simulink model "Citation"  (Simulink 10.1)
settings: Solver=ode5  StartTime=0.0  StopTime=inf  FixedStep=0.01  RelTol=1e-3  EnableMultiTasking=on
values from neighbouring files (symbols this model uses):
  S = 12.9900    (= 12.99)    [FTFC.m]
  Vw915 = 0    [initcit.m]
  winddir = 45*(pi/180)    (= 0.785398163397)    [initcit.m]
  x0 = []    [cessnac550_3d_sfnc.m]    (also in sfunxyz.m)
undefined symbols (not defined in the file or in its folder): chord, cv1, cv2, cv3, cv4, deltagmax1, deltagmax2, deltagmax3, deltagmax4, Deng, ealphag, ealphas, g0, hDME, hGS, kt1, kt2, kt3, lh, massinit, matbuaf, matdaf, matdam, matdbbf, matdeaf, matdgaf, matdqaf, matduaf, matdwaw, matedhr, mateif, matelhr, matemhr, matemv1, matemv2, matemve, matetam, mateuaf, matfaaf, matfaxl, matff, matibaf, matibmh, matipaf, matipmh, matiraf, matiuaf, matiwaf, matlaf, matlam, matleaf, matleam, matlgaf, matlqaf, matluaf, matmaaf, matmaam, matmaf, matmam, matmbbf ... (+74)
undefined symbols (not defined in the file): matibb
libraries: simulink x12, vrlib x1
(part 3 of 5)

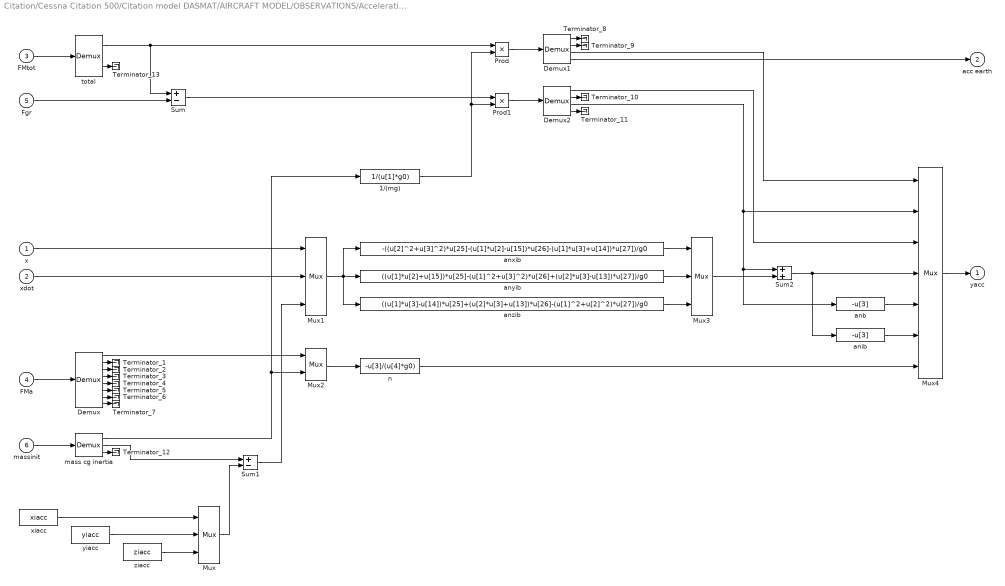
== system Citation/Cessna Citation 500/Citation model DASMAT/AIRCRAFT MODEL/OBSERVATIONS/Acceleration ==
  x : Inport
  xdot : Inport  Port=2
  FMtot : Inport  Port=3
  FMa : Inport  Port=4
  Fgr : Inport  Port=5
  massinit : Inport  Port=6
  1/(mg) : Fcn  Expr=1/(u[1]*g0)
  Demux : Demux  Outputs=[3 3 3 3 3 3 3 3]
      settings: DisplayOption=none
  Demux1 : Demux  Outputs=[3 3 3 3]
      settings: DisplayOption=none
  Demux2 : Demux  Outputs=[3 3 3 3]
      settings: DisplayOption=none
  Mux : Mux  Inputs=3
  Mux1 : Mux  Inputs=[12 12 3]
  Mux2 : Mux  Inputs=[3 1]
  Mux3 : Mux  Inputs=3
  Mux4 : Mux  Inputs=[3 3 3 3 1 1 1]
  Prod : Product  InputSameDT=on  SaturateOnIntegerOverflow=on  OutDataTypeStr=Inherit: Same as first input
  Prod1 : Product  InputSameDT=on  SaturateOnIntegerOverflow=on  OutDataTypeStr=Inherit: Same as first input
  Sum : Sum  Inputs=+-  InputSameDT=on  SaturateOnIntegerOverflow=on  OutDataTypeStr=Inherit: Same as first input
  Sum1 : Sum  Inputs=+-  InputSameDT=on  SaturateOnIntegerOverflow=on  OutDataTypeStr=Inherit: Same as first input
  Sum2 : Sum  InputSameDT=on  SaturateOnIntegerOverflow=on  OutDataTypeStr=Inherit: Same as first input
  Terminator_{1..13} (13 alike) : Terminator
  anb : Fcn  Expr=-u[3]
  anib : Fcn  Expr=-u[3]
  anxib : Fcn  Expr=-((u[2]^2+u[3]^2)*u[25]-(u[1]*u[2]-u[15])*u[26]-(u[1]*u[3]+u[14])*u[27])/g0
  anyib : Fcn  Expr=((u[1]*u[2]+u[15])*u[25]-(u[1]^2+u[3]^2)*u[26]+(u[2]*u[3]-u[13])*u[27])/g0
  anzib : Fcn  Expr=((u[1]*u[3]-u[14])*u[25]+(u[2]*u[3]+u[13])*u[26]-(u[1]^2+u[2]^2)*u[27])/g0
  mass cg inertia : Demux  Outputs=[1 3 4]
      settings: DisplayOption=none
  n : Fcn  Expr=-u[3]/(u[4]*g0)
  total : Demux  Outputs=[12 12]
      settings: DisplayOption=none
  xiacc : Constant  Value=xiacc
  yiacc : Constant  Value=yiacc
  ziacc : Constant  Value=ziacc
  yacc : Outport
  acc earth : Outport  Port=2
  wires:
  total/2 -> Terminator_13/1
  mass cg inertia/3 -> Terminator_12/1
  Demux2/4 -> Terminator_11/1
  Demux2/2 -> Terminator_10/1
  Demux1/2 -> Terminator_9/1
  Demux1/1 -> Terminator_8/1
  Demux/8 -> Terminator_7/1
  Demux/7 -> Terminator_6/1
  Demux/6 -> Terminator_5/1
  Demux/5 -> Terminator_4/1
  Demux/4 -> Terminator_3/1
  Demux/3 -> Terminator_2/1
  Demux/2 -> Terminator_1/1
  Mux4/1 -> yacc/1
  anb/1 -> Mux4/5
  Sum1/1 -> Mux1/3
  x/1 -> Mux1/1
  xdot/1 -> Mux1/2
  mass cg inertia/2 -> Sum1/1
  anzib/1 -> Mux3/3
  anxib/1 -> Mux3/1
  anyib/1 -> Mux3/2
  Mux2/1 -> n/1
  massinit/1 -> mass cg inertia/1
  xiacc/1 -> Mux/1
  yiacc/1 -> Mux/2
  ziacc/1 -> Mux/3
  1/(mg)/1 -> Prod1/2, Prod/2
  Sum/1 -> Prod1/1
  Mux1/1 -> anxib/1, anzib/1, anyib/1
  mass cg inertia/1 -> Mux2/2, 1/(mg)/1
  Mux/1 -> Sum1/2
  Mux3/1 -> Sum2/2
  Sum2/1 -> anib/1, Mux4/4
  FMa/1 -> Demux/1
  Fgr/1 -> Sum/2
  anib/1 -> Mux4/6
  n/1 -> Mux4/7
  total/1 -> Sum/1, Prod/1
  FMtot/1 -> total/1
  Demux/1 -> Mux2/1
  Demux2/3 -> Mux4/2, Sum2/1, anb/1
  Demux1/3 -> Mux4/1
  Prod/1 -> Demux1/1
  Demux2/1 -> Mux4/3
  Prod1/1 -> Demux2/1
  Demux1/4 -> acc earth/1

== system Citation/Cessna Citation 500/Citation model DASMAT/AIRCRAFT MODEL/OBSERVATIONS/Energy ==
  x : Inport
  xdot : Inport  Port=2
  yatm : Inport  Port=3
  Mux : Mux  Inputs=[12 12 8]
  Mux1 : Mux  Inputs=2
  spec energy : Fcn  Expr=u[10]+(u[4]*u[4])/(2*u[28])
  spec power : Fcn  Expr=u[22]+(u[4]*u[16])/u[28]
  ys : Outport
  wires:
  spec power/1 -> Mux1/2
  spec energy/1 -> Mux1/1
  x/1 -> Mux/1
  xdot/1 -> Mux/2
  Mux1/1 -> ys/1
  yatm/1 -> Mux/3
  Mux/1 -> spec power/1, spec energy/1

== system Citation/Cessna Citation 500/Citation model DASMAT/AIRCRAFT MODEL/OBSERVATIONS/Flight-Path ==
  x : Inport
  xdot : Inport  Port=2
  yuvw : Inport  Port=3
  acc earth : Inport  Port=4
  Demux : Demux  Outputs=[3 3 3 3]
      settings: DisplayOption=none
  Mux : Mux  Inputs=[12 12 3 3]
  Mux1 : Mux  Inputs=[30 1 1]
  Mux2 : Mux  Inputs=17
  Terminator11 : Terminator
  Terminator12 : Terminator
  Terminator13 : Terminator
  Vground : Fcn  Expr=sqrt(u[23]*u[23]+u[24]*u[24]+u[22]*u[22])
  bank angle : Fcn  Expr=asin(sin(u[7])*cos(u[8]))
  chi : Fcn  Expr=atan2(u[26],u[25])
  chidot : Fcn  Expr=(u[25]*u[29]*g0-u[28]*g0*u[26])/(u[4]*u[4]-u[27]*u[27])
  chimagn : Fcn  Expr=0
  chitrue : Fcn  Expr=atan2(u[24],u[23])
  chitruedot : Fcn  Expr=(u[23]*u[29]*g0-u[28]*g0*u[24])/(u[31]*u[31]-u[22]*u[22])
  flightpath acc : Fcn  Expr=u[16]/g0
  gamma : Fcn  Expr=asin(-u[27]/u[4])
  gammadot : Fcn  Expr=(-u[4]*u[30]*g0+u[16]*u[27])/(u[4]*sqrt(u[4]*u[4]-u[27]*u[27]))
  gammatrue : Fcn  Expr=asin(u[22]/u[31])
  gammatruedot : Fcn  Expr=(u[31]*u[32]*g0-u[16]*u[22])/(u[31]*sqrt(u[31]*u[31]-u[22]*u[22]))
  gsdev : Fcn  Expr=atan2(u[10]-hGS,sqrt((xGS-u[11])*(xGS-u[11])+(yGS-u[12])*(yGS-u[12]))) - 3*pi/180
  locdev : Fcn  Expr=psiLOC - atan2(yLOC-u[12],xLOC-u[11])
  psimagn : Fcn  Expr=0
  range : Fcn  Expr=sqrt((u[11]-xDME)*(u[11]-xDME)+(u[12]-yDME)*(u[12]-yDME)+(u[10]-hDME)*(u[10]-hDME))
  vertical acc : Fcn  Expr=-u[30]
  yfp : Outport
  wires:
  Demux/3 -> Terminator13/1
  Demux/2 -> Terminator12/1
  Demux/1 -> Terminator11/1
  vertical acc/1 -> Mux1/3, Mux2/16
  Mux1/1 -> gammatruedot/1, chitruedot/1, gammatrue/1, chitrue/1
  Vground/1 -> Mux1/2, Mux2/15
  xdot/1 -> Mux/2
  Demux/4 -> Mux/3
  acc earth/1 -> Mux/4
  yuvw/1 -> Demux/1
  chi/1 -> Mux2/2
  Mux2/1 -> yfp/1
  gamma/1 -> Mux2/1
  gammadot/1 -> Mux2/3
  chidot/1 -> Mux2/4
  gammatrue/1 -> Mux2/5
  chitrue/1 -> Mux2/6
  gammatruedot/1 -> Mux2/7
  flightpath acc/1 -> Mux2/17
  range/1 -> Mux2/14
  locdev/1 -> Mux2/13
  gsdev/1 -> Mux2/12
  bank angle/1 -> Mux2/11
  psimagn/1 -> Mux2/10
  chimagn/1 -> Mux2/9
  chitruedot/1 -> Mux2/8
  x/1 -> Mux/1
  Mux/1 -> Mux1/1, gammadot/1, chi/1, gamma/1, chidot/1, gsdev/1, locdev/1, range/1, Vground/1, vertical acc/1, flightpath acc/1, bank angle/1, psimagn/1, chimagn/1

== system Citation/Cessna Citation 500/Citation model DASMAT/AIRCRAFT MODEL/WIND/TURBULENCE/Logarithmic Wind model ==
  In1 : Inport
  He Selector : Selector  InputPortWidth=12  IndexOptions=Index vector (dialog)  Indices=[10]  OutputSizes=1
  Logarithmic Wind model : Subsystem
  Mux : Mux  Inputs=3
  Out1 : Outport
  wires:
  In1/1 -> He Selector/1
  Mux/1 -> Out1/1
  Logarithmic Wind model/1(uwind) -> Mux/1  "uwind"
  Logarithmic Wind model/2(vwind) -> Mux/2  "vwind"
  Logarithmic Wind model/3(wwind) -> Mux/3  "wwind"
  He Selector/1 -> Logarithmic Wind model/1(he)

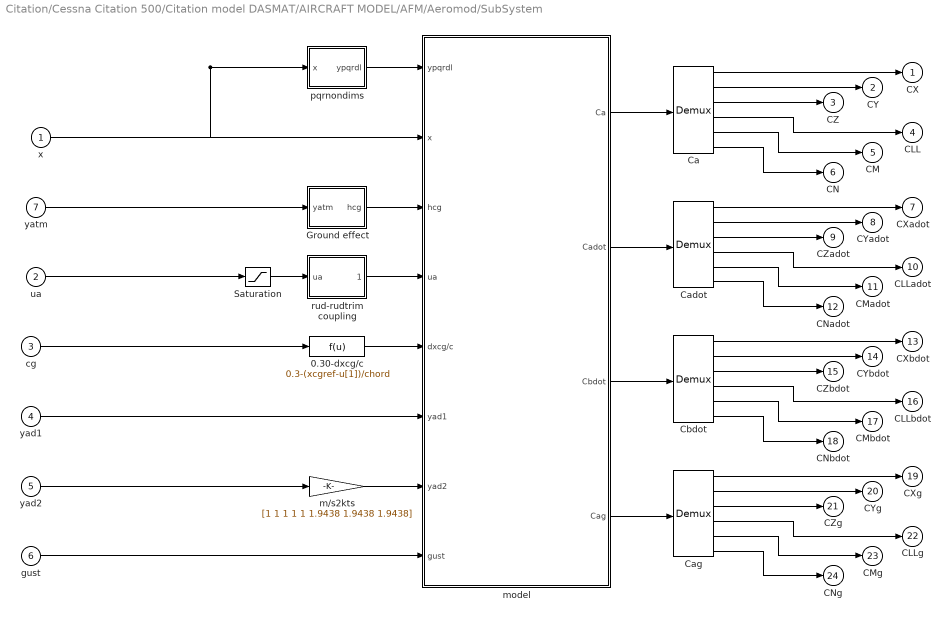
== system Citation/Cessna Citation 500/Citation model DASMAT/AIRCRAFT MODEL/AFM/Aeromod/SubSystem ==
  x : Inport
  ua : Inport  Port=2
  cg : Inport  Port=3
  yad1 : Inport  Port=4
  yad2 : Inport  Port=5
  gust : Inport  Port=6
  yatm : Inport  Port=7
  0.30-dxcg/c : Fcn  Expr=0.3-(xcgref-u[1])/chord
  Ca : Demux  Outputs=6
      settings: DisplayOption=none
  Cadot : Demux  Outputs=6
      settings: DisplayOption=none
  Cag : Demux  Outputs=6
      settings: DisplayOption=none
  Cbdot : Demux  Outputs=6
      settings: DisplayOption=none
  Ground effect : Subsystem
  Saturation : Saturate  UpperLimit="[ 15  37  22  15  20  10 40 180/pi]*pi/180"  LowerLimit="[-20 -37 -22 -15 -20 -10 0  0]*pi/180"
  m/s2kts : Gain  Gain=[1 1 1 1 1 1.9438 1.9438 1.9438]  SaturateOnIntegerOverflow=on  OutDataTypeStr=Inherit: Same as input  ParamDataTypeStr=Inherit: Same as input
  model : Subsystem
  pqrnondims : Subsystem
  rud-rudtrim coupling : Subsystem
  CX : Outport
  CY : Outport  Port=2
  CZ : Outport  Port=3
  CLL : Outport  Port=4
  CM : Outport  Port=5
  CN : Outport  Port=6
  CXadot : Outport  Port=7
  CYadot : Outport  Port=8
  CZadot : Outport  Port=9
  CLLadot : Outport  Port=10
  CMadot : Outport  Port=11
  CNadot : Outport  Port=12
  CXbdot : Outport  Port=13
  CYbdot : Outport  Port=14
  CZbdot : Outport  Port=15
  CLLbdot : Outport  Port=16
  CMbdot : Outport  Port=17
  CNbdot : Outport  Port=18
  CXg : Outport  Port=19
  CYg : Outport  Port=20
  CZg : Outport  Port=21
  CLLg : Outport  Port=22
  CMg : Outport  Port=23
  CNg : Outport  Port=24
  wires:
  yad2/1 -> m/s2kts/1
  m/s2kts/1 -> model/7(yad2)
  Saturation/1 -> rud-rudtrim coupling/1(ua)
  model/4(Cag) -> Cag/1
  model/3(Cbdot) -> Cbdot/1
  Cbdot/2 -> CYbdot/1
  Cbdot/1 -> CXbdot/1
  Cbdot/3 -> CZbdot/1
  Cbdot/4 -> CLLbdot/1
  Cbdot/5 -> CMbdot/1
  Cbdot/6 -> CNbdot/1
  Cag/6 -> CNg/1
  Cag/5 -> CMg/1
  Cag/4 -> CLLg/1
  Cag/3 -> CZg/1
  Cag/1 -> CXg/1
  Cag/2 -> CYg/1
  model/2(Cadot) -> Cadot/1
  Cadot/2 -> CYadot/1
  Cadot/1 -> CXadot/1
  Cadot/3 -> CZadot/1
  Cadot/4 -> CLLadot/1
  Cadot/5 -> CMadot/1
  Cadot/6 -> CNadot/1
  Ca/6 -> CN/1
  Ca/5 -> CM/1
  Ca/4 -> CLL/1
  Ca/3 -> CZ/1
  Ca/1 -> CX/1
  Ca/2 -> CY/1
  model/1(Ca) -> Ca/1
  yad1/1 -> model/6(yad1)
  gust/1 -> model/8(gust)
  cg/1 -> 0.30-dxcg/c/1
  ua/1 -> Saturation/1
  x/1 -> pqrnondims/1(x), model/2(x)
  0.30-dxcg/c/1 -> model/5(dxcg/c)
  Ground effect/1(hcg) -> model/3(hcg)
  rud-rudtrim coupling/1(ua coupled) -> model/4(ua)
  pqrnondims/1(ypqrdl) -> model/1(ypqrdl)
  yatm/1 -> Ground effect/1(yatm)

== system Citation/Cessna Citation 500/Citation model DASMAT/AIRCRAFT MODEL/AFM/FMaerodims/dims ==
  note: X,Y,Z
  FM/length : Inport
  Demux : Demux  Outputs=[12 3 3 3 3]
      settings: DisplayOption=none
  LL,M,N air : Gain  Gain=[span chord span]  SaturateOnIntegerOverflow=on  OutDataTypeStr=Inherit: Same as input  ParamDataTypeStr=Inherit: Same as input
  LL,M,N body : Gain  Gain=[span chord span]  SaturateOnIntegerOverflow=on  OutDataTypeStr=Inherit: Same as input  ParamDataTypeStr=Inherit: Same as input
  LL,M,N earth : Gain  Gain=[span chord span]  SaturateOnIntegerOverflow=on  OutDataTypeStr=Inherit: Same as input  ParamDataTypeStr=Inherit: Same as input
  LL,M,N stab : Gain  Gain=[span chord span]  SaturateOnIntegerOverflow=on  OutDataTypeStr=Inherit: Same as input  ParamDataTypeStr=Inherit: Same as input
  Mux : Mux  Inputs=[12 3 3 3 3]
  FM : Outport
  wires:
  LL,M,N earth/1 -> Mux/5
  Demux/5 -> LL,M,N earth/1
  LL,M,N body/1 -> Mux/4
  LL,M,N stab/1 -> Mux/3
  LL,M,N air/1 -> Mux/2
  Demux/1 -> Mux/1
  Demux/2 -> LL,M,N air/1
  Demux/3 -> LL,M,N stab/1
  Demux/4 -> LL,M,N body/1
  Mux/1 -> FM/1
  FM/length/1 -> Demux/1

== system Citation/Cessna Citation 500/Citation model DASMAT/AIRCRAFT MODEL/AFM/FMaerodims/dims1 ==
  note: X,Y,Z
  F FM/length : Inport
  Demux : Demux  Outputs=[12 3 3 3 3]
      settings: DisplayOption=none
  LL,M,N air : Gain  Gain=[span chord span]  SaturateOnIntegerOverflow=on  OutDataTypeStr=Inherit: Same as input  ParamDataTypeStr=Inherit: Same as input
  LL,M,N body : Gain  Gain=[span chord span]  SaturateOnIntegerOverflow=on  OutDataTypeStr=Inherit: Same as input  ParamDataTypeStr=Inherit: Same as input
  LL,M,N earth : Gain  Gain=[span chord span]  SaturateOnIntegerOverflow=on  OutDataTypeStr=Inherit: Same as input  ParamDataTypeStr=Inherit: Same as input
  LL,M,N stab : Gain  Gain=[span chord span]  SaturateOnIntegerOverflow=on  OutDataTypeStr=Inherit: Same as input  ParamDataTypeStr=Inherit: Same as input
  Mux : Mux  Inputs=[12 3 3 3 3]
  FM : Outport
  wires:
  F FM/length/1 -> Demux/1
  Mux/1 -> FM/1
  Demux/4 -> LL,M,N body/1
  Demux/3 -> LL,M,N stab/1
  Demux/2 -> LL,M,N air/1
  Demux/1 -> Mux/1
  LL,M,N air/1 -> Mux/2
  LL,M,N stab/1 -> Mux/3
  LL,M,N body/1 -> Mux/4
  Demux/5 -> LL,M,N earth/1
  LL,M,N earth/1 -> Mux/5

== system Citation/Cessna Citation 500/Citation model DASMAT/AIRCRAFT MODEL/AFM/FMaerodims/dims2 ==
  note: X,Y,Z
  F FM/length : Inport
  Demux : Demux  Outputs=[12 3 3 3 3]
      settings: DisplayOption=none
  LL,M,N air : Gain  Gain=[span chord span]  SaturateOnIntegerOverflow=on  OutDataTypeStr=Inherit: Same as input  ParamDataTypeStr=Inherit: Same as input
  LL,M,N body : Gain  Gain=[span chord span]  SaturateOnIntegerOverflow=on  OutDataTypeStr=Inherit: Same as input  ParamDataTypeStr=Inherit: Same as input
  LL,M,N earth : Gain  Gain=[span chord span]  SaturateOnIntegerOverflow=on  OutDataTypeStr=Inherit: Same as input  ParamDataTypeStr=Inherit: Same as input
  LL,M,N stab : Gain  Gain=[span chord span]  SaturateOnIntegerOverflow=on  OutDataTypeStr=Inherit: Same as input  ParamDataTypeStr=Inherit: Same as input
  Mux : Mux  Inputs=[12 3 3 3 3]
  FM : Outport
  wires:
  LL,M,N earth/1 -> Mux/5
  Demux/5 -> LL,M,N earth/1
  LL,M,N body/1 -> Mux/4
  LL,M,N stab/1 -> Mux/3
  LL,M,N air/1 -> Mux/2
  Demux/1 -> Mux/1
  Demux/2 -> LL,M,N air/1
  Demux/3 -> LL,M,N stab/1
  Demux/4 -> LL,M,N body/1
  Mux/1 -> FM/1
  F FM/length/1 -> Demux/1

== system Citation/Cessna Citation 500/Citation model DASMAT/AIRCRAFT MODEL/AFM/FMgustdims/dims ==
  note: X,Y,Z
  F M/length : Inport
  Demux : Demux  Outputs=[12 3 3 3 3]
      settings: DisplayOption=none
  LL,M,N air : Gain  Gain=[span chord span]  SaturateOnIntegerOverflow=on  OutDataTypeStr=Inherit: Same as input  ParamDataTypeStr=Inherit: Same as input
  LL,M,N body : Gain  Gain=[span chord span]  SaturateOnIntegerOverflow=on  OutDataTypeStr=Inherit: Same as input  ParamDataTypeStr=Inherit: Same as input
  LL,M,N earth : Gain  Gain=[span chord span]  SaturateOnIntegerOverflow=on  OutDataTypeStr=Inherit: Same as input  ParamDataTypeStr=Inherit: Same as input
  LL,M,N stab : Gain  Gain=[span chord span]  SaturateOnIntegerOverflow=on  OutDataTypeStr=Inherit: Same as input  ParamDataTypeStr=Inherit: Same as input
  Mux : Mux  Inputs=[12 3 3 3 3]
  FM : Outport
  wires:
  LL,M,N earth/1 -> Mux/5
  Demux/5 -> LL,M,N earth/1
  LL,M,N body/1 -> Mux/4
  LL,M,N stab/1 -> Mux/3
  LL,M,N air/1 -> Mux/2
  Demux/1 -> Mux/1
  Demux/2 -> LL,M,N air/1
  Demux/3 -> LL,M,N stab/1
  Demux/4 -> LL,M,N body/1
  Mux/1 -> FM/1
  F M/length/1 -> Demux/1

== system Citation/Cessna Citation 500/Citation model DASMAT/AIRCRAFT MODEL/EFM/Engmod/Citation eng_mod ==
  In1 : Inport
  Demux : Demux  Outputs=32
      settings: DisplayOption=none
  Mux : Mux  Inputs=6
  Mux1 : Mux  Inputs=2
  Subsystem1 : Subsystem
  Out1 : Outport
  ypp : Outport  Port=2
  wires:
  Subsystem1/4(MXt) -> Mux/4
  Subsystem1/3(Zt) -> Mux/3
  Subsystem1/2(Yt) -> Mux/2
  Subsystem1/1(Xt) -> Mux/1
  Subsystem1/6(MZt) -> Mux/6
  Subsystem1/5(MYt) -> Mux/5
  Mux/1 -> Out1/1
  In1/1 -> Demux/1
  Demux/1 -> Subsystem1/1(pbody)
  Demux/2 -> Subsystem1/2(qbody)
  Demux/3 -> Subsystem1/3(rbody)
  Demux/4 -> Subsystem1/4(VTAS)
  Demux/5 -> Subsystem1/5(alpha)
  Demux/6 -> Subsystem1/6(beta)
  Demux/7 -> Subsystem1/7(phi)
  Demux/8 -> Subsystem1/8(theta)
  Demux/9 -> Subsystem1/9(psi)
  Demux/10 -> Subsystem1/10(he)
  Demux/11 -> Subsystem1/11(xe)
  Demux/12 -> Subsystem1/12(ye)
  Demux/13 -> Subsystem1/13(ut1)
  Demux/14 -> Subsystem1/14(ut2)
  Demux/15 -> Subsystem1/15(pstat)
  Demux/16 -> Subsystem1/16(rho)
  Demux/17 -> Subsystem1/17(temp)
  Demux/18 -> Subsystem1/18(grav)
  Demux/19 -> Subsystem1/19(hpress)
  Demux/20 -> Subsystem1/20(hradio)
  Demux/21 -> Subsystem1/21(Hgeopot)
  Demux/22 -> Subsystem1/22(Vsound)
  Demux/23 -> Subsystem1/23(Mach)
  Demux/24 -> Subsystem1/24(qdyn)
  Demux/25 -> Subsystem1/25(Reynl)
  Demux/26 -> Subsystem1/26(qc)
  Demux/27 -> Subsystem1/27(qrel)
  Demux/28 -> Subsystem1/28(ptot)
  Demux/29 -> Subsystem1/29(temptot)
  Demux/30 -> Subsystem1/30(VEAS)
  Demux/31 -> Subsystem1/31(VCAS)
  Demux/32 -> Subsystem1/32(VIAS)
  Subsystem1/7(yppleft) -> Mux1/1
  Subsystem1/8(yppright) -> Mux1/2
  Mux1/1 -> ypp/1

== system Citation/Cessna Citation 500/Citation model DASMAT/AIRCRAFT MODEL/EQM/State Derivatives/Vabdot ==
  x : Inport
  ypqr : Inport  Port=2
  Ftot : Inport  Port=3
  Fadot : Inport  Port=4
  Fbdot : Inport  Port=5
  mass : Inport  Port=6
  wind : Inport  Port=7
  Mux1 : Mux  Inputs=3
  Prod : Product  InputSameDT=on  SaturateOnIntegerOverflow=on  OutDataTypeStr=Inherit: Same as first input
  Prod1 : Product  InputSameDT=on  SaturateOnIntegerOverflow=on  OutDataTypeStr=Inherit: Same as first input
  Sum : Sum  Inputs=+++  InputSameDT=on  SaturateOnIntegerOverflow=on  OutDataTypeStr=Inherit: Same as first input
  Vdot : Subsystem
  abdot : Subsystem
  winddot : Derivative
  Vabdot : Outport
  Ftot corrected : Outport  Port=2
  wires:
  wind/1 -> winddot/1, Vdot/5(wind), abdot/7(wind)
  winddot/1 -> abdot/8(winddot), Vdot/6(winddot)
  Vdot/1(Vdot) -> Mux1/1
  mass/1 -> Vdot/4(mass), abdot/6(mass)
  ypqr/1 -> Vdot/2(ypqr), abdot/2(ypqr)
  x/1 -> Vdot/1(x), abdot/1(x)
  abdot/1(adot) -> Vdot/7(adot), Prod/2, Mux1/2
  abdot/2(bdot) -> Vdot/8(bdot), Prod1/2, Mux1/3
  Fbdot/1 -> abdot/5(Fbdot), Prod1/1
  Fadot/1 -> abdot/4(Fadot), Prod/1
  Prod1/1 -> Sum/3
  Mux1/1 -> Vabdot/1
  Sum/1 -> Vdot/3(Ftot), Ftot corrected/1
  Prod/1 -> Sum/2
  Ftot/1 -> abdot/3(Ftot), Sum/1

== system Citation/Cessna Citation 500/Citation model DASMAT/AIRCRAFT MODEL/EQM/State Derivatives/eulerdot ==
  x : Inport
  Mux : Mux  Inputs=3
  phidot : Fcn  Expr=u[1]+tan(u[8])*(u[2]*sin(u[7])+u[3]*cos(u[7]))
  psidot : Fcn  Expr=(u[2]*sin(u[7])+u[3]*cos(u[7]))/cos(u[8])
  thetadot : Fcn  Expr=u[2]*cos(u[7])-u[3]*sin(u[7])
  eulerdot : Outport
  wires:
  x/1 -> phidot/1, psidot/1, thetadot/1
  Mux/1 -> eulerdot/1
  phidot/1 -> Mux/1
  thetadot/1 -> Mux/2
  psidot/1 -> Mux/3

== system Citation/Cessna Citation 500/Citation model DASMAT/AIRCRAFT MODEL/EQM/State Derivatives/hxydot ==
  yuvw : Inport
  wind : Inport  Port=2
  Demux : Demux  Outputs=[3 3 3 3]
      settings: DisplayOption=none
  Demux1 : Demux  Outputs=[3 3 3 3]
      settings: DisplayOption=none
  Mux : Mux  Inputs=[3 3]
  Mux1 : Mux  Inputs=3
  Terminator_{1..6} (6 alike) : Terminator
  hedot : Fcn  Expr=-(u[3]+u[6])
  xedot : Fcn  Expr=u[1]+u[4]
  yedot : Fcn  Expr=u[2]+u[5]
  hxydot : Outport
  wires:
  Demux1/3 -> Terminator_6/1
  Demux1/2 -> Terminator_5/1
  Demux1/1 -> Terminator_4/1
  Demux/3 -> Terminator_3/1
  Demux/2 -> Terminator_2/1
  Demux/1 -> Terminator_1/1
  wind/1 -> Demux1/1
  Demux1/4 -> Mux/2
  yedot/1 -> Mux1/3
  xedot/1 -> Mux1/2
  hedot/1 -> Mux1/1  "hedot"
  Mux1/1 -> hxydot/1
  Mux/1 -> hedot/1, yedot/1, xedot/1
  yuvw/1 -> Demux/1
  Demux/4 -> Mux/1

== system Citation/Cessna Citation 500/Citation model DASMAT/AIRCRAFT MODEL/EQM/State Derivatives/mass properties ==
  massinit : Inport
  GAMMA : Fcn  Expr=u[1]*u[3]-u[4]*u[4]
  Mux : Mux  Inputs=[4 1]
  Mux1 : Mux  Inputs=9
  Terminator_1 : Terminator
  c1 : Fcn  Expr=((u[2]-u[3])*u[3]-u[4]*u[4])/u[5]
  c2 : Fcn  Expr=(u[1]-u[2]+u[3])*u[4]/u[5]
  c3 : Fcn  Expr=u[3]/u[5]
  c4 : Fcn  Expr=u[4]/u[5]
  c5 : Fcn  Expr=(u[3]-u[1])/u[2]
  c6 : Fcn  Expr=u[4]/u[2]
  c7 : Fcn  Expr=1/u[2]
  c8 : Fcn  Expr=((u[1]-u[2])*u[1]+u[4]*u[4])/u[5]
  c9 : Fcn  Expr=u[1]/u[5]
  mass cg inertia : Demux  Outputs=[1 3 4]
      settings: DisplayOption=none
  mass : Outport
  inertia : Outport  Port=2
  wires:
  mass cg inertia/2 -> Terminator_1/1
  massinit/1 -> mass cg inertia/1
  mass cg inertia/1 -> mass/1
  mass cg inertia/3 -> GAMMA/1, Mux/1
  GAMMA/1 -> Mux/2
  c1/1 -> Mux1/1
  c2/1 -> Mux1/2
  c3/1 -> Mux1/3
  c4/1 -> Mux1/4
  c5/1 -> Mux1/5
  c6/1 -> Mux1/6
  c7/1 -> Mux1/7
  c8/1 -> Mux1/8
  c9/1 -> Mux1/9
  Mux1/1 -> inertia/1
  Mux/1 -> c2/1, c3/1, c4/1, c5/1, c6/1, c7/1, c8/1, c9/1, c1/1

== system Citation/Cessna Citation 500/Citation model DASMAT/AIRCRAFT MODEL/EQM/State Derivatives/pqrdot ==
  ypqr : Inport
  Mtot : Inport  Port=2
  Madot : Inport  Port=3
  Mbdot : Inport  Port=4
  inertia : Inport  Port=5
  Vabdot : Inport  Port=6
  Demux : Demux  Outputs=3
      settings: DisplayOption=none
  Demux1 : Demux  Outputs=[3 3 3 3]
      settings: DisplayOption=none
  Demux2 : Demux  Outputs=[3 3 3 3]
      settings: DisplayOption=none
  Mux : Mux  Inputs=[3 3 9]
  Mux1 : Mux  Inputs=3
  Prod : Product  InputSameDT=on  SaturateOnIntegerOverflow=on  OutDataTypeStr=Inherit: Same as first input
  Prod1 : Product  InputSameDT=on  SaturateOnIntegerOverflow=on  OutDataTypeStr=Inherit: Same as first input
  Sum : Sum  Inputs=+++  InputSameDT=on  SaturateOnIntegerOverflow=on  OutDataTypeStr=Inherit: Same as first input
  Terminator_{1..7} (7 alike) : Terminator
  pdot : Fcn  Expr=(u[7]*u[3]+u[8]*u[1])*u[2]+u[9]*u[4]+u[10]*u[6]
  qdot : Fcn  Expr=u[11]*u[1]*u[3]-u[12]*(u[1]^2-u[3]^2)+u[13]*u[5]
  rdot : Fcn  Expr=(u[14]*u[1]-u[8]*u[3])*u[2]+u[10]*u[4]+u[15]*u[6]
  pqrdot : Outport
  Mtot corrected : Outport  Port=2
  wires:
  Demux2/4 -> Terminator_7/1
  Demux2/2 -> Terminator_6/1
  Demux2/1 -> Terminator_5/1
  Demux1/4 -> Terminator_4/1
  Demux1/2 -> Terminator_3/1
  Demux1/1 -> Terminator_2/1
  Demux/1 -> Terminator_1/1
  Demux2/3 -> Mux/2
  Demux1/3 -> Mux/1
  inertia/1 -> Mux/3
  qdot/1 -> Mux1/2
  pdot/1 -> Mux1/1
  Mux/1 -> pdot/1, rdot/1, qdot/1
  Mux1/1 -> pqrdot/1
  ypqr/1 -> Demux1/1
  Demux/3 -> Prod1/2
  Demux/2 -> Prod/2
  Mbdot/1 -> Prod1/1
  Madot/1 -> Prod/1
  Mtot/1 -> Sum/1
  Vabdot/1 -> Demux/1
  Prod1/1 -> Sum/3
  Sum/1 -> Demux2/1, Mtot corrected/1
  Prod/1 -> Sum/2
  rdot/1 -> Mux1/3

== system Citation/Cessna Citation 500/Citation model DASMAT/AIRCRAFT MODEL/EQM/State Derivatives/states transformation ==
  x : Inport
  1/V : Fcn  Expr=1/u[4]
  Demux : Demux  Outputs=[3 3 3 3]
      settings: DisplayOption=none
  Mux : Mux  Inputs=[12 1 1 1]
  Mux1 : Mux  Inputs=[12 1 1 1]
  Mux2 : Mux  Inputs=3
  Mux3 : Mux  Inputs=[3 3 3 3 12]
  Prod{,1..4} (5 alike) : Product  InputSameDT=on  SaturateOnIntegerOverflow=on  OutDataTypeStr=Inherit: Same as first input
  Terminator_{1..8} (8 alike) : Terminator
  Vab transformation : S-Function  FunctionName=ac_axes  Parameters=0  SFunctionDeploymentMode=off  EnableBusSupport=off
  b/2V : Fcn  Expr=span/(2*u[4])
  b/2V1 : Fcn  Expr=span/(2*u[4])
  c/V : Fcn  Expr=chord/u[4]
  pqr transformation : S-Function  FunctionName=ac_axes  Parameters=2  SFunctionDeploymentMode=off  EnableBusSupport=off
  states : Demux  Outputs=12
      settings: DisplayOption=none
  zero : Constant  Value=0
  ypqr : Outport
  yuvw : Outport  Port=2
  ydl : Outport  Port=3
  wires:
  states/12 -> Terminator_8/1
  states/11 -> Terminator_7/1
  states/10 -> Terminator_6/1
  states/9 -> Terminator_5/1
  states/8 -> Terminator_4/1
  states/7 -> Terminator_3/1
  states/6 -> Terminator_2/1
  states/5 -> Terminator_1/1
  states/3 -> Mux/4
  states/2 -> Mux/3
  states/1 -> Mux/2
  Mux/1 -> pqr transformation/1
  Mux1/1 -> Vab transformation/1
  zero/1 -> Mux1/3, Mux1/4
  states/4 -> Mux1/2
  c/V/1 -> Mux2/2
  b/2V1/1 -> Mux2/3
  b/2V/1 -> Mux2/1
  Demux/1 -> Prod/1
  Demux/2 -> Prod1/1
  Demux/3 -> Prod2/1
  Demux/4 -> Prod3/1
  1/V/1 -> Prod4/2
  pqr transformation/1 -> Demux/1, ypqr/1
  Vab transformation/1 -> Prod4/1, yuvw/1
  Mux2/1 -> Prod1/2, Prod/2, Prod2/2, Prod3/2
  Prod/1 -> Mux3/1
  Prod1/1 -> Mux3/2
  Prod2/1 -> Mux3/3
  Prod3/1 -> Mux3/4
  Prod4/1 -> Mux3/5
  Mux3/1 -> ydl/1
  x/1 -> Mux/1, Mux1/1, b/2V/1, b/2V1/1, c/V/1, 1/V/1, states/1

== system Citation/Cessna Citation 500/Citation model DASMAT/AIRCRAFT MODEL/LANDING GEAR/Landing Gear model/Correct for terrain elevation ==
  x : Inport
  terr elev : Inport  Port=2
  Demux : Demux  Outputs=[9 1 2]
      settings: DisplayOption=none
  Mux : Mux  Inputs=3
  terrain elevation corr : Sum  Inputs=-+|  SaturateOnIntegerOverflow=on
  x corrected : Outport
  wires:
  x/1 -> Demux/1
  Demux/1 -> Mux/1
  Demux/3 -> Mux/3
  Mux/1 -> x corrected/1
  Demux/2 -> terrain elevation corr/2
  terr elev/1 -> terrain elevation corr/1
  terrain elevation corr/1 -> Mux/2

== system Citation/Cessna Citation 500/Citation model DASMAT/AIRCRAFT MODEL/LANDING GEAR/Landing Gear model/Left Main Gear ==
  Inputs : Inport
  Axes Transformation Heading attached vertical axis to body axis : Subsystem
  Calculation of the Moments : Subsystem
  Demux : Demux  Outputs=[6 2 5]
      settings: DisplayOption=none
  FS Side Force : Constant  Value=0
  FV Vertical Force : Subsystem
  Fmu Longitudinal Force : Fcn  Expr=u[1]*murol
  Mux : Mux  Inputs=3
  Mux1 : Mux  Inputs=2
  Terminator : Terminator
  Terminator1 : Terminator
  FX FY FZ : Outport
  L M N : Outport  Port=2
  wires:
  Fmu Longitudinal Force/1 -> Mux/1
  FS Side Force/1 -> Mux/2
  FV Vertical Force/1(Out1) -> Fmu Longitudinal Force/1, Mux/3
  Calculation of the Moments/1(L M N) -> L M N/1
  Inputs/1 -> FV Vertical Force/1(In1), Demux/1
  Demux/1 -> Terminator/1
  Demux/3 -> Terminator1/1
  Mux1/1 -> Axes Transformation Heading attached vertical axis to body axis/1(Fmu FS FV phi theta)
  Mux/1 -> Mux1/1
  Demux/2 -> Mux1/2  "phi theta"
  Axes Transformation Heading attached vertical axis to body axis/1(FX FY FZ) -> FX FY FZ/1, Calculation of the Moments/1(FX FY FZ)

== system Citation/Cessna Citation 500/Citation model DASMAT/AIRCRAFT MODEL/LANDING GEAR/Landing Gear model/Nose Gear ==
  Inputs : Inport
  Axes Transformation Heading attached vertical axis to body axis : Subsystem
  Calculation of the Moments : Subsystem
  Demux : Demux  Outputs=[6 2 5]
      settings: DisplayOption=none
  F Vertical Force : Subsystem
  FS Side Force : Constant  Value=0
  Fmu Longitudinal Force : Fcn  Expr=u[1]*murol
  Mux : Mux  Inputs=3
  Mux1 : Mux  Inputs=2
  Terminator : Terminator
  Terminator1 : Terminator
  FX FY FZ : Outport
  L M N : Outport  Port=2
  wires:
  Fmu Longitudinal Force/1 -> Mux/1
  FS Side Force/1 -> Mux/2
  F Vertical Force/1(Out1) -> Fmu Longitudinal Force/1, Mux/3
  Calculation of the Moments/1(L M N) -> L M N/1
  Inputs/1 -> F Vertical Force/1(In1), Demux/1
  Demux/1 -> Terminator/1
  Demux/3 -> Terminator1/1
  Mux1/1 -> Axes Transformation Heading attached vertical axis to body axis/1(Fmu FS FV phi theta)
  Mux/1 -> Mux1/1
  Demux/2 -> Mux1/2  "phi theta"
  Axes Transformation Heading attached vertical axis to body axis/1(FX FY FZ) -> FX FY FZ/1, Calculation of the Moments/1(FX FY FZ)

== system Citation/Cessna Citation 500/Citation model DASMAT/AIRCRAFT MODEL/LANDING GEAR/Landing Gear model/Right Main Gear ==
  Inputs : Inport
  Axes Transformation Heading attached vertical axis to body axis : Subsystem
  Calculation of the Moments : Subsystem
  Demux : Demux  Outputs=[6 2 5]
      settings: DisplayOption=none
  FS Side Force : Constant  Value=0
  FV Vertical Force : Subsystem
  Fmu Longitudinal Force : Fcn  Expr=u[1]*murol
  Mux : Mux  Inputs=3
  Mux1 : Mux  Inputs=2
  Terminator : Terminator
  Terminator1 : Terminator
  FX FY FZ : Outport
  L M N : Outport  Port=2
  wires:
  Fmu Longitudinal Force/1 -> Mux/1
  FS Side Force/1 -> Mux/2
  FV Vertical Force/1(Out1) -> Fmu Longitudinal Force/1, Mux/3
  Calculation of the Moments/1(L M N) -> L M N/1
  Inputs/1 -> FV Vertical Force/1(In1), Demux/1
  Demux/1 -> Terminator/1
  Demux/3 -> Terminator1/1
  Mux1/1 -> Axes Transformation Heading attached vertical axis to body axis/1(Fmu FS FV phi theta)
  Mux/1 -> Mux1/1
  Demux/2 -> Mux1/2  "phi theta"
  Axes Transformation Heading attached vertical axis to body axis/1(FX FY FZ) -> FX FY FZ/1, Calculation of the Moments/1(FX FY FZ)

== system Citation/Cessna Citation 500/Citation model DASMAT/AIRCRAFT MODEL/LANDING GEAR/Landing Gear model/Tail Scraper ==
  Inputs : Inport
  Axes Transformation Heading attached vertical axis to body axis : Subsystem
  Calculation of the Moments : Subsystem
  Demux : Demux  Outputs=[6 2 5]
      settings: DisplayOption=none
  FS Side Force : Constant  Value=0
  FV Vertical Force : Subsystem
  Fmu : Constant  Value=0
  Mux : Mux  Inputs=3
  Mux1 : Mux  Inputs=2
  Terminator : Terminator
  Terminator1 : Terminator
  FX FY FZ : Outport
  L M N : Outport  Port=2
  wires:
  Fmu/1 -> Mux/1
  FS Side Force/1 -> Mux/2
  Calculation of the Moments/1(L M N) -> L M N/1
  Inputs/1 -> FV Vertical Force/1(In1), Demux/1
  Demux/1 -> Terminator/1
  Demux/3 -> Terminator1/1
  Mux1/1 -> Axes Transformation Heading attached vertical axis to body axis/1(Fmu FS FV phi theta)
  Mux/1 -> Mux1/1
  Demux/2 -> Mux1/2  "phi theta"
  Axes Transformation Heading attached vertical axis to body axis/1(FX FY FZ) -> FX FY FZ/1, Calculation of the Moments/1(FX FY FZ)
  FV Vertical Force/1(Out1) -> Mux/3

== system Citation/Cessna Citation 500/Citation model DASMAT/AIRCRAFT MODEL/WIND/TURBULENCE/Logarithmic Wind model/Logarithmic Wind model ==
  note: winddir output deleted
      | you can calculate it yourself
      | from uvw, you lazy bastard
  note: runway elevation
      | correction deleted,
      | is all relative to sea level
  he : Inport
  Constant : Constant  Value=0
  Mux : Mux  Inputs=2
  Product : Product  InputSameDT=on  SaturateOnIntegerOverflow=on  OutDataTypeStr=Inherit: Same as first input
  Switch : Switch  Threshold=300  SaturateOnIntegerOverflow=on  InputSameDT=on
  Vwind above 300m : Fcn  Expr=1.637
  Vwind below 300m : Fcn  Expr=(0.43*log10(u)+0.572)
  Vwind915 : Subsystem
  Windddirection : Subsystem
  uwind earth axis : Fcn  Expr=cos(u[1])*u[2]
  vwind earth axis : Fcn  Expr=sin(u[1])*u[2]
  uwind : Outport
  vwind : Outport  Port=2
  wwind : Outport  Port=3
  wires:
  Vwind above 300m/1 -> Switch/1
  Vwind below 300m/1 -> Switch/3
  Constant/1 -> wwind/1
  he/1 -> Switch/2, Vwind above 300m/1, Vwind below 300m/1
  Switch/1 -> Product/2
  Vwind915/1(Out1) -> Product/1
  Product/1 -> Mux/2
  Windddirection/1(Out1) -> Mux/1
  uwind earth axis/1 -> uwind/1
  vwind earth axis/1 -> vwind/1
  Mux/1 -> uwind earth axis/1, vwind earth axis/1

== system Citation/Cessna Citation 500/Citation model DASMAT/AIRCRAFT MODEL/AFM/Aeromod/SubSystem/Ground effect ==
  yatm : Inport
  Sat : Saturate  UpperLimit=21  LowerLimit=-inf
  radio alt selector : Selector  IndexOptions=Index vector (dialog)  Indices=[6]  OutputSizes=1
  hcg : Outport
  wires:
  radio alt selector/1 -> Sat/1
  Sat/1 -> hcg/1
  yatm/1 -> radio alt selector/1

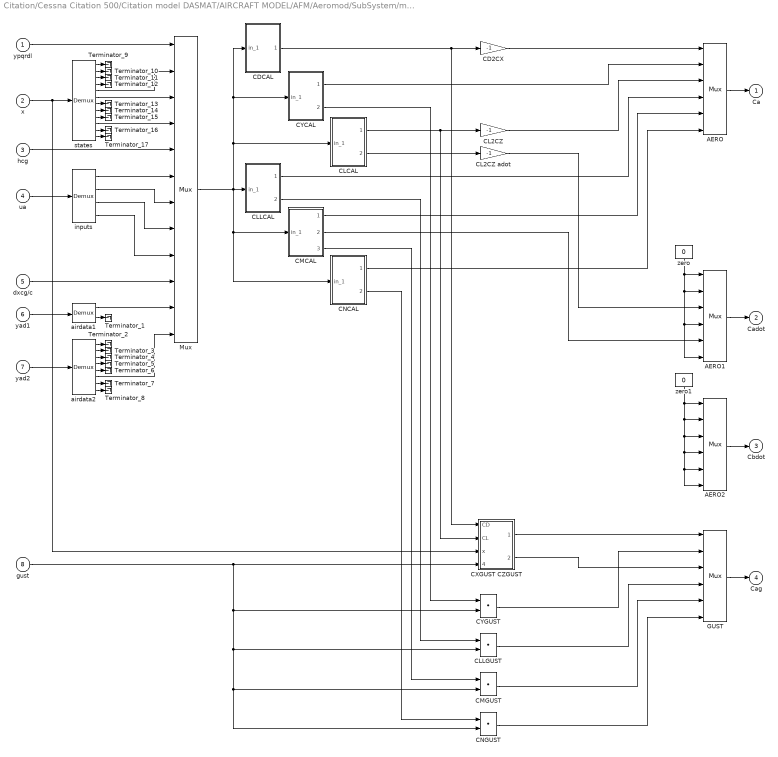
== system Citation/Cessna Citation 500/Citation model DASMAT/AIRCRAFT MODEL/AFM/Aeromod/SubSystem/model ==
  ypqrdl : Inport
  x : Inport  Port=2
  hcg : Inport  Port=3
  ua : Inport  Port=4
  dxcg/c : Inport  Port=5
  yad1 : Inport  Port=6
  yad2 : Inport  Port=7
  gust : Inport  Port=8
  AERO : Mux  Inputs=6
  AERO1 : Mux  Inputs=6
  AERO2 : Mux  Inputs=6
  CD2CX : Gain  Gain=-1  SaturateOnIntegerOverflow=on  OutDataTypeStr=Inherit: Same as input  ParamDataTypeStr=Inherit: Same as input
  CDCAL : Subsystem
  CL2CZ : Gain  Gain=-1  SaturateOnIntegerOverflow=on  OutDataTypeStr=Inherit: Same as input  ParamDataTypeStr=Inherit: Same as input
  CL2CZ adot : Gain  Gain=-1  SaturateOnIntegerOverflow=on  OutDataTypeStr=Inherit: Same as input  ParamDataTypeStr=Inherit: Same as input
  CLCAL : Subsystem
  CLLCAL : Subsystem
  CLLGUST : DotProduct  InputSameDT=on  OutDataTypeStr=Inherit: Inherit via internal rule
  CMCAL : Subsystem
  CMGUST : DotProduct  InputSameDT=on  OutDataTypeStr=Inherit: Inherit via internal rule
  CNCAL : Subsystem
  CNGUST : DotProduct  InputSameDT=on  OutDataTypeStr=Inherit: Inherit via internal rule
  CXGUST CZGUST : Subsystem
  CYCAL : Subsystem
  CYGUST : DotProduct  InputSameDT=on  OutDataTypeStr=Inherit: Inherit via internal rule
  GUST : Mux  Inputs=6
  Mux : Mux  Inputs=[3 1 1 1 1 3 3 1 1 1 1 1]
  Terminator_{1..17} (17 alike) : Terminator
  airdata1 : Demux  Outputs=2
      settings: DisplayOption=none
  airdata2 : Demux  Outputs=8
      settings: DisplayOption=none
  inputs : Demux  Outputs=[3 3 1 1]
      settings: DisplayOption=none
  states : Demux  Outputs=12
      settings: DisplayOption=none
  zero : Constant  Value=0
  zero1 : Constant  Value=0
  Ca : Outport
  Cadot : Outport  Port=2
  Cbdot : Outport  Port=3
  Cag : Outport  Port=4
  wires:
  states/12 -> Terminator_17/1
  states/11 -> Terminator_16/1
  states/9 -> Terminator_15/1
  states/8 -> Terminator_14/1
  states/7 -> Terminator_13/1
  states/4 -> Terminator_12/1
  states/3 -> Terminator_11/1
  states/2 -> Terminator_10/1
  states/1 -> Terminator_9/1
  airdata2/8 -> Terminator_8/1
  airdata2/7 -> Terminator_7/1
  airdata2/5 -> Terminator_6/1
  airdata2/4 -> Terminator_5/1
  airdata2/3 -> Terminator_4/1
  airdata2/2 -> Terminator_3/1
  airdata2/1 -> Terminator_2/1
  airdata1/2 -> Terminator_1/1
  gust/1 -> CYGUST/2, CLLGUST/2, CMGUST/2, CNGUST/2, CXGUST CZGUST/4(gust)
  x/1 -> CXGUST CZGUST/3(x), states/1
  airdata1/1 -> Mux/11
  CDCAL/1(out_1) -> CXGUST CZGUST/1(CD), CD2CX/1
  CNCAL/2("out_2 ") -> CNGUST/1
  CMCAL/3("out_3 ") -> CMGUST/1
  CMCAL/2(out_2) -> AERO1/5
  CMCAL/1(out_1) -> AERO/5
  CNCAL/1(out_1) -> AERO/6
  CLLCAL/2(out_2) -> CLLGUST/1
  CLLCAL/1(out_1) -> AERO/4
  CLCAL/2(out_2) -> CL2CZ adot/1
  CYCAL/2(out_2) -> CYGUST/1
  CYCAL/1(out_1) -> AERO/2
  CL2CZ adot/1 -> AERO1/3
  CNGUST/1 -> GUST/6
  CLLGUST/1 -> GUST/4
  CMGUST/1 -> GUST/5
  CYGUST/1 -> GUST/2
  CLCAL/1(out_1) -> CXGUST CZGUST/2(CL), CL2CZ/1
  CL2CZ/1 -> AERO/3
  CD2CX/1 -> AERO/1
  airdata2/6 -> Mux/12
  CXGUST CZGUST/2("out_2 ") -> GUST/3
  GUST/1 -> Cag/1
  AERO/1 -> Ca/1
  Mux/1 -> CMCAL/1(in_1), CNCAL/1(in_1), CLCAL/1(in_1), CYCAL/1(in_1), CDCAL/1(in_1), CLLCAL/1(in_1)
  CXGUST CZGUST/1("out_1 ") -> GUST/1
  yad2/1 -> airdata2/1
  inputs/3 -> Mux/8
  hcg/1 -> Mux/5
  ua/1 -> inputs/1
  yad1/1 -> airdata1/1
  dxcg/c/1 -> Mux/10
  states/6 -> Mux/3
  states/10 -> Mux/4
  ypqrdl/1 -> Mux/1
  inputs/1 -> Mux/6
  states/5 -> Mux/2
  inputs/4 -> Mux/9
  inputs/2 -> Mux/7
  AERO1/1 -> Cadot/1
  zero/1 -> AERO1/4, AERO1/6, AERO1/2, AERO1/1
  zero1/1 -> AERO2/1, AERO2/2, AERO2/3, AERO2/4, AERO2/5, AERO2/6
  AERO2/1 -> Cbdot/1

== system Citation/Cessna Citation 500/Citation model DASMAT/AIRCRAFT MODEL/AFM/Aeromod/SubSystem/pqrnondims ==
  x : Inport
  Demux : Demux  Outputs=[3 3 3 3]
      settings: DisplayOption=none
  Mux : Mux  Inputs=[12 1 1 1]
  Mux1 : Mux  Inputs=3
  Prod : Product  InputSameDT=on  SaturateOnIntegerOverflow=on  OutDataTypeStr=Inherit: Same as first input
  Terminator_{1..12} (12 alike) : Terminator
  b/2V : Fcn  Expr=span/(2*u[4])
  b/2V1 : Fcn  Expr=span/(2*u[4])
  c/V : Fcn  Expr=chord/u[4]
  pqr transformation : S-Function  FunctionName=ac_axes  Parameters=2  SFunctionDeploymentMode=off  EnableBusSupport=off
  states : Demux  Outputs=12
      settings: DisplayOption=none
  ypqrdl : Outport
  wires:
  states/12 -> Terminator_12/1
  states/11 -> Terminator_11/1
  states/10 -> Terminator_10/1
  states/9 -> Terminator_9/1
  states/8 -> Terminator_8/1
  states/7 -> Terminator_7/1
  states/6 -> Terminator_6/1
  states/5 -> Terminator_5/1
  states/4 -> Terminator_4/1
  Demux/4 -> Terminator_3/1
  Demux/3 -> Terminator_2/1
  Demux/1 -> Terminator_1/1
  Mux/1 -> pqr transformation/1
  states/1 -> Mux/2
  states/2 -> Mux/3
  states/3 -> Mux/4
  Prod/1 -> ypqrdl/1
  Mux1/1 -> Prod/2
  x/1 -> states/1, b/2V/1, b/2V1/1, c/V/1, Mux/1
  b/2V/1 -> Mux1/1
  b/2V1/1 -> Mux1/3
  c/V/1 -> Mux1/2
  pqr transformation/1 -> Demux/1
  Demux/2 -> Prod/1

== system Citation/Cessna Citation 500/Citation model DASMAT/AIRCRAFT MODEL/AFM/Aeromod/SubSystem/rud-rudtrim coupling ==
  ua : Inport
  Demux : Demux  Outputs=[3 1 1 1 2]
      settings: DisplayOption=none
  Mux : Mux  Inputs=[3 1 1 1 2]
  Terminator_1 : Terminator
  rud-rudtrim coupled : Fcn  Expr=u[6]+0.536*u[3]
  ua coupled : Outport
  wires:
  Demux/4 -> Terminator_1/1
  Mux/1 -> ua coupled/1
  Demux/5 -> Mux/5
  Demux/3 -> Mux/3
  Demux/2 -> Mux/2
  rud-rudtrim coupled/1 -> Mux/4
  Demux/1 -> Mux/1
  ua/1 -> rud-rudtrim coupled/1, Demux/1

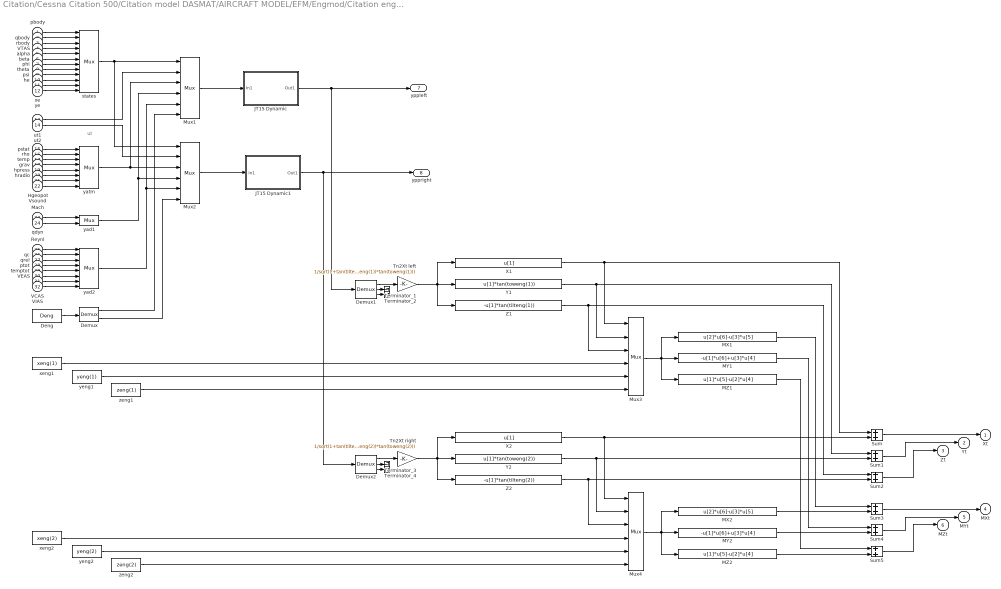
== system Citation/Cessna Citation 500/Citation model DASMAT/AIRCRAFT MODEL/EFM/Engmod/Citation eng_mod/Subsystem1 ==
  note: ut
  pbody : Inport
  qbody : Inport  Port=2
  rbody : Inport  Port=3
  VTAS : Inport  Port=4
  alpha : Inport  Port=5
  beta : Inport  Port=6
  phi : Inport  Port=7
  theta : Inport  Port=8
  psi : Inport  Port=9
  he : Inport  Port=10
  xe : Inport  Port=11
  ye : Inport  Port=12
  ut1 : Inport  Port=13
  ut2 : Inport  Port=14
  pstat : Inport  Port=15
  rho : Inport  Port=16
  temp : Inport  Port=17
  grav : Inport  Port=18
  hpress : Inport  Port=19
  hradio : Inport  Port=20
  Hgeopot : Inport  Port=21
  Vsound : Inport  Port=22
  Mach : Inport  Port=23
  qdyn : Inport  Port=24
  Reynl : Inport  Port=25
  qc : Inport  Port=26
  qrel : Inport  Port=27
  ptot : Inport  Port=28
  temptot : Inport  Port=29
  VEAS : Inport  Port=30
  VCAS : Inport  Port=31
  VIAS : Inport  Port=32
  Demux : Demux  Outputs=2
      settings: DisplayOption=none
  Demux1 : Demux  Outputs=[1 1 -1]
      settings: DisplayOption=none
  Demux2 : Demux  Outputs=[1 1 -1]
      settings: DisplayOption=none
  Deng : Constant  Value=Deng
  JT15 Dynamic : Subsystem
  JT15 Dynamic1 : Subsystem
  MX1 : Fcn  Expr=u[2]*u[6]-u[3]*u[5]
  MX2 : Fcn  Expr=u[2]*u[6]-u[3]*u[5]
  MY1 : Fcn  Expr=-u[1]*u[6]+u[3]*u[4]
  MY2 : Fcn  Expr=-u[1]*u[6]+u[3]*u[4]
  MZ1 : Fcn  Expr=u[1]*u[5]-u[2]*u[4]
  MZ2 : Fcn  Expr=u[1]*u[5]-u[2]*u[4]
  Mux1 : Mux  Inputs=[12 1 8 2 8 1]
  Mux2 : Mux  Inputs=[12 1 8 2 8 1]
  Mux3 : Mux  Inputs=6
  Mux4 : Mux  Inputs=6
  Sum{,1..5} (6 alike) : Sum  InputSameDT=on  SaturateOnIntegerOverflow=on  OutDataTypeStr=Inherit: Same as first input
  Terminator_{1..4} (4 alike) : Terminator
  Tn2Xt left : Gain  Gain=1/sqrt(1+tan(tilteng(1))*tan(tilteng(1))+tan(toweng(1))*tan(toweng(1)))  SaturateOnIntegerOverflow=on  OutDataTypeStr=Inherit: Same as input  ParamDataTypeStr=Inherit: Same as input
  Tn2Xt right : Gain  Gain=1/sqrt(1+tan(tilteng(2))*tan(tilteng(2))+tan(toweng(2))*tan(toweng(2)))  SaturateOnIntegerOverflow=on  OutDataTypeStr=Inherit: Same as input  ParamDataTypeStr=Inherit: Same as input
  X1 : Fcn  Expr=u[1]
  X2 : Fcn  Expr=u[1]
  Y1 : Fcn  Expr=u[1]*tan(toweng(1))
  Y2 : Fcn  Expr=u[1]*tan(toweng(2))
  Z1 : Fcn  Expr=-u[1]*tan(tilteng(1))
  Z2 : Fcn  Expr=-u[1]*tan(tilteng(2))
  states : Mux  Inputs=12
  xeng1 : Constant  Value=xeng(1)
  xeng2 : Constant  Value=xeng(2)
  yad1 : Mux  Inputs=2
  yad2 : Mux  Inputs=8
  yatm : Mux  Inputs=8
  yeng1 : Constant  Value=yeng(1)
  yeng2 : Constant  Value=yeng(2)
  zeng1 : Constant  Value=zeng(1)
  zeng2 : Constant  Value=zeng(2)
  Xt : Outport
  Yt : Outport  Port=2
  Zt : Outport  Port=3
  MXt : Outport  Port=4
  MYt : Outport  Port=5
  MZt : Outport  Port=6
  yppleft : Outport  Port=7
  yppright : Outport  Port=8
  wires:
  grav/1 -> yatm/4
  hradio/1 -> yatm/6
  temp/1 -> yatm/3
  hpress/1 -> yatm/5
  Hgeopot/1 -> yatm/7
  rho/1 -> yatm/2
  pstat/1 -> yatm/1
  pbody/1 -> states/1
  qbody/1 -> states/2
  phi/1 -> states/7
  alpha/1 -> states/5
  rbody/1 -> states/3
  theta/1 -> states/8
  beta/1 -> states/6
  VTAS/1 -> states/4
  psi/1 -> states/9
  he/1 -> states/10
  xe/1 -> states/11
  ye/1 -> states/12
  ptot/1 -> yad2/4
  VEAS/1 -> yad2/6
  VIAS/1 -> yad2/8
  qrel/1 -> yad2/3
  temptot/1 -> yad2/5
  VCAS/1 -> yad2/7
  qc/1 -> yad2/2
  Reynl/1 -> yad2/1
  qdyn/1 -> yad1/2
  Mux1/1 -> JT15 Dynamic/1(In1)
  Mux2/1 -> JT15 Dynamic1/1(In1)
  Tn2Xt left/1 -> Y1/1, X1/1, Z1/1
  xeng1/1 -> Mux3/4
  yeng1/1 -> Mux3/5
  zeng1/1 -> Mux3/6
  Mux3/1 -> MY1/1, MX1/1, MZ1/1
  zeng2/1 -> Mux4/6
  yeng2/1 -> Mux4/5
  xeng2/1 -> Mux4/4
  Tn2Xt right/1 -> Y2/1, Z2/1, X2/1
  MZ2/1 -> Sum5/2
  MY2/1 -> Sum4/2
  MX2/1 -> Sum3/2
  Mux4/1 -> MY2/1, MZ2/1, MX2/1
  MZ1/1 -> Sum5/1
  MY1/1 -> Sum4/1
  MX1/1 -> Sum3/1
  Y2/1 -> Sum1/2, Mux4/2
  X2/1 -> Sum/2, Mux4/1
  X1/1 -> Sum/1, Mux3/1
  Z1/1 -> Sum2/1, Mux3/3
  Y1/1 -> Sum1/1, Mux3/2
  Z2/1 -> Sum2/2, Mux4/3
  Sum/1 -> Xt/1
  Sum1/1 -> Yt/1
  Sum2/1 -> Zt/1
  Sum3/1 -> MXt/1
  Sum4/1 -> MYt/1
  Sum5/1 -> MZt/1
  ut1/1 -> Mux1/2
  yad1/1 -> Mux1/4, Mux2/4
  yad2/1 -> Mux1/5, Mux2/5
  yatm/1 -> Mux2/3, Mux1/3
  ut2/1 -> Mux2/2
  states/1 -> Mux1/1, Mux2/1
  Demux1/1 -> Tn2Xt left/1
  Demux2/1 -> Tn2Xt right/1
  Vsound/1 -> yatm/8
  Mach/1 -> yad1/1
  Deng/1 -> Demux/1
  Demux/1 -> Mux1/6
  Demux/2 -> Mux2/6
  Demux1/2 -> Terminator_1/1
  Demux1/3 -> Terminator_2/1
  Demux2/2 -> Terminator_3/1
  Demux2/3 -> Terminator_4/1
  JT15 Dynamic/1(Out1) -> Demux1/1, yppleft/1
  JT15 Dynamic1/1(Out1) -> Demux2/1, yppright/1

== system Citation/Cessna Citation 500/Citation model DASMAT/AIRCRAFT MODEL/EQM/State Derivatives/Vabdot/Vdot ==
  x : Inport
  ypqr : Inport  Port=2
  Ftot : Inport  Port=3
  mass : Inport  Port=4
  wind : Inport  Port=5
  winddot : Inport  Port=6
  adot : Inport  Port=7
  bdot : Inport  Port=8
  Demux{,1..3} (4 alike) : Demux  Outputs=[3 3 3 3]
      settings: DisplayOption=none
  Mux2 : Mux  Inputs=[3 3 3 3 1 1 1 1 1]
  Terminator_{1..22} (22 alike) : Terminator
  VTASdot : Fcn  Expr=u[1]/u[17]-(u[10]+(u[5]-u[15]*cos(u[14]))*u[9]-(u[6]-u[16])*u[8])
  states : Demux  Outputs=12
      settings: DisplayOption=none
  Vdot : Outport
  wires:
  states/12 -> Terminator_22/1
  states/11 -> Terminator_21/1
  states/10 -> Terminator_20/1
  states/9 -> Terminator_19/1
  states/8 -> Terminator_18/1
  states/7 -> Terminator_17/1
  states/5 -> Terminator_16/1
  states/3 -> Terminator_15/1
  states/2 -> Terminator_14/1
  states/1 -> Terminator_13/1
  Demux3/4 -> Terminator_12/1
  Demux3/3 -> Terminator_11/1
  Demux3/2 -> Terminator_10/1
  Demux2/4 -> Terminator_9/1
  Demux2/3 -> Terminator_8/1
  Demux2/2 -> Terminator_7/1
  Demux1/4 -> Terminator_6/1
  Demux1/3 -> Terminator_5/1
  Demux1/2 -> Terminator_4/1
  Demux/4 -> Terminator_3/1
  Demux/3 -> Terminator_2/1
  Demux/2 -> Terminator_1/1
  Demux3/1 -> Mux2/4
  Mux2/1 -> VTASdot/1
  winddot/1 -> Demux3/1
  states/6 -> Mux2/6
  adot/1 -> Mux2/7
  mass/1 -> Mux2/9
  bdot/1 -> Mux2/8
  Demux2/1 -> Mux2/3
  states/4 -> Mux2/5
  wind/1 -> Demux2/1
  Ftot/1 -> Demux/1
  Demux/1 -> Mux2/1
  Demux1/1 -> Mux2/2
  ypqr/1 -> Demux1/1
  x/1 -> states/1
  VTASdot/1 -> Vdot/1

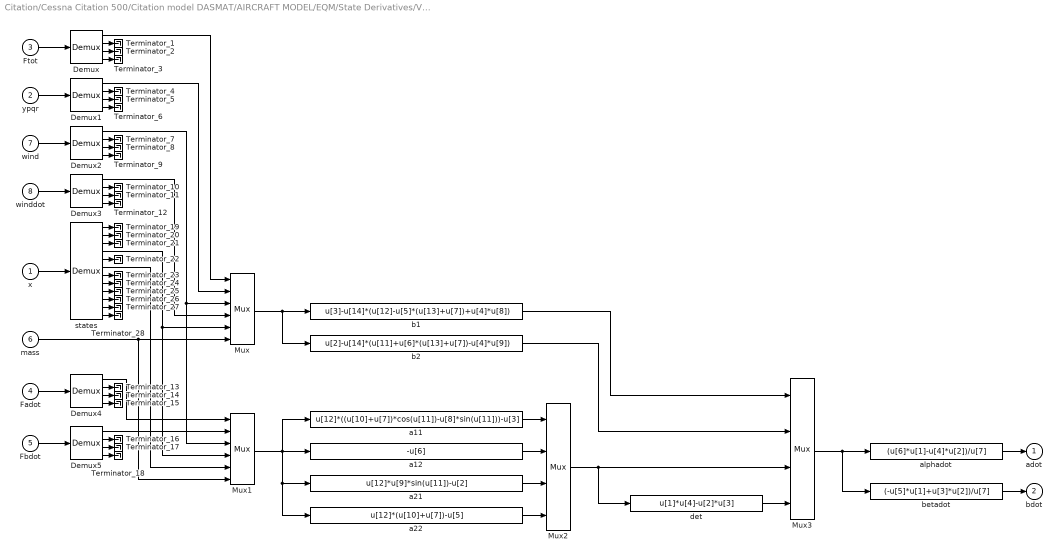
== system Citation/Cessna Citation 500/Citation model DASMAT/AIRCRAFT MODEL/EQM/State Derivatives/Vabdot/abdot ==
  x : Inport
  ypqr : Inport  Port=2
  Ftot : Inport  Port=3
  Fadot : Inport  Port=4
  Fbdot : Inport  Port=5
  mass : Inport  Port=6
  wind : Inport  Port=7
  winddot : Inport  Port=8
  Demux{,1..5} (6 alike) : Demux  Outputs=[3 3 3 3]
      settings: DisplayOption=none
  Mux : Mux  Inputs=[3 3 3 3 1 1]
  Mux1 : Mux  Inputs=[3 3 3 1 1 1]
  Mux2 : Mux
  Mux3 : Mux  Inputs=[1 1 4 1]
  Terminator_{1..28} (28 alike) : Terminator
  a11 : Fcn  Expr=u[12]*((u[10]+u[7])*cos(u[11])-u[8]*sin(u[11]))-u[3]
  a12 : Fcn  Expr=-u[6]
  a21 : Fcn  Expr=u[12]*u[9]*sin(u[11])-u[2]
  a22 : Fcn  Expr=u[12]*(u[10]+u[7])-u[5]
  alphadot : Fcn  Expr=(u[6]*u[1]-u[4]*u[2])/u[7]
  b1 : Fcn  Expr=u[3]-u[14]*(u[12]-u[5]*(u[13]+u[7])+u[4]*u[8])
  b2 : Fcn  Expr=u[2]-u[14]*(u[11]+u[6]*(u[13]+u[7])-u[4]*u[9])
  betadot : Fcn  Expr=(-u[5]*u[1]+u[3]*u[2])/u[7]
  det : Fcn  Expr=u[1]*u[4]-u[2]*u[3]
  states : Demux  Outputs=12
      settings: DisplayOption=none
  adot : Outport
  bdot : Outport  Port=2
  wires:
  states/12 -> Terminator_28/1
  states/11 -> Terminator_27/1
  states/10 -> Terminator_26/1
  states/9 -> Terminator_25/1
  states/8 -> Terminator_24/1
  states/7 -> Terminator_23/1
  states/5 -> Terminator_22/1
  states/3 -> Terminator_21/1
  states/2 -> Terminator_20/1
  states/1 -> Terminator_19/1
  Demux5/4 -> Terminator_18/1
  Demux5/3 -> Terminator_17/1
  Demux5/2 -> Terminator_16/1
  Demux4/4 -> Terminator_15/1
  Demux4/3 -> Terminator_14/1
  Demux4/2 -> Terminator_13/1
  Demux3/4 -> Terminator_12/1
  Demux3/3 -> Terminator_11/1
  Demux3/2 -> Terminator_10/1
  Demux2/4 -> Terminator_9/1
  Demux2/3 -> Terminator_8/1
  Demux2/2 -> Terminator_7/1
  Demux1/4 -> Terminator_6/1
  Demux1/3 -> Terminator_5/1
  Demux1/2 -> Terminator_4/1
  Demux/4 -> Terminator_3/1
  Demux/3 -> Terminator_2/1
  Demux/2 -> Terminator_1/1
  states/4 -> Mux/5, Mux1/4
  Demux2/1 -> Mux/3, Mux1/3
  Demux3/1 -> Mux/4
  winddot/1 -> Demux3/1
  states/6 -> Mux1/5
  Mux3/1 -> betadot/1, alphadot/1
  Mux/1 -> b2/1, b1/1
  b1/1 -> Mux3/1
  b2/1 -> Mux3/2
  det/1 -> Mux3/4
  Mux2/1 -> det/1, Mux3/3
  a22/1 -> Mux2/4
  a21/1 -> Mux2/3
  a12/1 -> Mux2/2
  a11/1 -> Mux2/1
  x/1 -> states/1
  Demux5/1 -> Mux1/2
  alphadot/1 -> adot/1
  betadot/1 -> bdot/1
  ypqr/1 -> Demux1/1
  Demux1/1 -> Mux/2
  Demux/1 -> Mux/1
  Ftot/1 -> Demux/1
  Demux4/1 -> Mux1/1
  Fbdot/1 -> Demux5/1
  Fadot/1 -> Demux4/1
  wind/1 -> Demux2/1
  mass/1 -> Mux1/6, Mux/6
  Mux1/1 -> a21/1, a22/1, a11/1, a12/1

== system Citation/Cessna Citation 500/Citation model DASMAT/AIRCRAFT MODEL/LANDING GEAR/Landing Gear model/Left Main Gear/Axes Transformation Heading attached vertical axis to body axis ==
  Fmu FS FV phi theta : Inport
  FX : Fcn  Expr=-cos(u[5])*u[1]+0*u[2]+sin(u[5])*u[3]
  FY : Fcn  Expr=-sin(u[5])*sin(u[4])*u[1]-cos(u[4])*u[2]-cos(u[5])*sin(u[4])*u[3]
  FZ : Fcn  Expr=-sin(u[5])*cos(u[4])*u[1]+sin(u[4])*u[2]-cos(u[5])*cos(u[4])*u[3]
  Mux1 : Mux  Inputs=3
  FX FY FZ : Outport
  wires:
  Fmu FS FV phi theta/1 -> FX/1, FY/1, FZ/1
  FX/1 -> Mux1/1
  FY/1 -> Mux1/2
  FZ/1 -> Mux1/3
  Mux1/1 -> FX FY FZ/1

== system Citation/Cessna Citation 500/Citation model DASMAT/AIRCRAFT MODEL/LANDING GEAR/Landing Gear model/Left Main Gear/Calculation of the Moments ==
  FX FY FZ : Inport
  L : Fcn  Expr=0*u[1]-zl1*u[2]+yl1*u[3]
  M : Fcn  Expr=zl1*u[1]+0*u[2]-xl1*u[3]
  Mux2 : Mux  Inputs=3
  N : Fcn  Expr=-yl1*u[1]+xl1*u[2]+0*u[3]
  L M N : Outport
  wires:
  L/1 -> Mux2/1
  M/1 -> Mux2/2
  N/1 -> Mux2/3
  FX FY FZ/1 -> M/1, L/1, N/1
  Mux2/1 -> L M N/1

== system Citation/Cessna Citation 500/Citation model DASMAT/AIRCRAFT MODEL/LANDING GEAR/Landing Gear model/Left Main Gear/FV Vertical Force ==
  In1 : Inport
  B : Fcn  Expr=(u[2]/kt1)-u[1]-deltagmax1
  C : Fcn  Expr=(deltagmax1/kt1)*(P1+u[2]-(kt1*u[1]))
  FD damping force : Fcn  Expr=cv1*u[1]
  FV : Fcn  Expr=kt1*(u[1]-u[2])
  FV No ground contact : Constant  Value=0
  Mux1 : Mux  Inputs=2
  Mux2 : Mux  Inputs=2
  Mux3 : Mux  Inputs=2
  No negative  Strut deflection : Saturate  UpperLimit=inf  LowerLimit=0
  Prevent Earth  from pulling a/c when FD>FV : Saturate  UpperLimit=inf  LowerLimit=0
  Strut deflection : Fcn  Expr=0.5*(-u[1]-sqrt(u[1]*u[1]+4*u[2]))
  Switch1 : Switch  SaturateOnIntegerOverflow=on  InputSameDT=on
  deltag : Fcn  Expr=zl1-u[10]-xl1*sin(u[8])+yl1*sin(u[7])
  deltagdot : Fcn  Expr=-u[13]-xl1*u[2]*cos(u[8])+yl1*u[1]*cos(u[7])
  Out1 : Outport
  wires:
  In1/1 -> deltag/1, deltagdot/1
  deltagdot/1 -> FD damping force/1
  Strut deflection/1 -> No negative  Strut deflection/1
  FD damping force/1 -> Mux1/2
  Mux1/1 -> B/1, C/1
  B/1 -> Mux2/1
  C/1 -> Mux2/2
  Mux2/1 -> Strut deflection/1
  Mux3/1 -> FV/1
  No negative  Strut deflection/1 -> Mux3/2
  deltag/1 -> Mux1/1, Mux3/1, Switch1/2
  FV/1 -> Prevent Earth  from pulling a/c when FD>FV/1
  FV No ground contact/1 -> Switch1/3
  Prevent Earth  from pulling a/c when FD>FV/1 -> Switch1/1
  Switch1/1 -> Out1/1

== system Citation/Cessna Citation 500/Citation model DASMAT/AIRCRAFT MODEL/LANDING GEAR/Landing Gear model/Nose Gear/Axes Transformation Heading attached vertical axis to body axis ==
  Fmu FS FV phi theta : Inport
  FX : Fcn  Expr=-cos(u[5])*u[1]+0*u[2]+sin(u[5])*u[3]
  FY : Fcn  Expr=-sin(u[5])*sin(u[4])*u[1]-cos(u[4])*u[2]-cos(u[5])*sin(u[4])*u[3]
  FZ : Fcn  Expr=-sin(u[5])*cos(u[4])*u[1]+sin(u[4])*u[2]-cos(u[5])*cos(u[4])*u[3]
  Mux1 : Mux  Inputs=3
  FX FY FZ : Outport
  wires:
  Fmu FS FV phi theta/1 -> FX/1, FY/1, FZ/1
  FX/1 -> Mux1/1
  FY/1 -> Mux1/2
  FZ/1 -> Mux1/3
  Mux1/1 -> FX FY FZ/1

== system Citation/Cessna Citation 500/Citation model DASMAT/AIRCRAFT MODEL/LANDING GEAR/Landing Gear model/Nose Gear/Calculation of the Moments ==
  FX FY FZ : Inport
  L : Fcn  Expr=0*u[1]-zl3*u[2]+yl3*u[3]
  M : Fcn  Expr=zl3*u[1]+0*u[2]-xl3*u[3]
  Mux2 : Mux  Inputs=3
  N : Fcn  Expr=-yl3*u[1]+xl3*u[2]+0*u[3]
  L M N : Outport
  wires:
  L/1 -> Mux2/1
  M/1 -> Mux2/2
  N/1 -> Mux2/3
  FX FY FZ/1 -> M/1, L/1, N/1
  Mux2/1 -> L M N/1

== system Citation/Cessna Citation 500/Citation model DASMAT/AIRCRAFT MODEL/LANDING GEAR/Landing Gear model/Nose Gear/F Vertical Force ==
  In1 : Inport
  B : Fcn  Expr=(u[2]/kt3)-u[1]-deltagmax3
  C : Fcn  Expr=(deltagmax3/kt3)*(P3+u[2]-(kt3*u[1]))
  FD damping force : Fcn  Expr=cv3*u[1]
  FV : Fcn  Expr=kt3*(u[1]-u[2])
  FV No ground contact : Constant  Value=0
  Mux1 : Mux  Inputs=2
  Mux2 : Mux  Inputs=2
  Mux3 : Mux  Inputs=2
  No negative  Strut deflection : Saturate  UpperLimit=inf  LowerLimit=0
  Prevent Earth  from pulling a/c when FD>FV : Saturate  UpperLimit=inf  LowerLimit=0
  Strut deflection : Fcn  Expr=0.5*(-u[1]-sqrt(u[1]*u[1]+4*u[2]))
  Switch1 : Switch  SaturateOnIntegerOverflow=on  InputSameDT=on
  deltag : Fcn  Expr=zl3-u[10]-xl3*sin(u[8])+yl3*sin(u[7])
  deltagdot : Fcn  Expr=-u[13]-xl3*u[2]*cos(u[8])+yl3*u[1]*cos(u[7])
  Out1 : Outport
  wires:
  In1/1 -> deltag/1, deltagdot/1
  deltagdot/1 -> FD damping force/1
  Strut deflection/1 -> No negative  Strut deflection/1
  FD damping force/1 -> Mux1/2
  Mux1/1 -> B/1, C/1
  B/1 -> Mux2/1
  C/1 -> Mux2/2
  Mux2/1 -> Strut deflection/1
  Mux3/1 -> FV/1
  No negative  Strut deflection/1 -> Mux3/2
  deltag/1 -> Mux1/1, Mux3/1, Switch1/2
  FV/1 -> Prevent Earth  from pulling a/c when FD>FV/1
  FV No ground contact/1 -> Switch1/3
  Prevent Earth  from pulling a/c when FD>FV/1 -> Switch1/1
  Switch1/1 -> Out1/1
